simulink model "IRSensor"  (Simulink 8.7)
settings: Solver=VariableStepAuto  StartTime=0.0  StopTime=10.0  RelTol=1e-3
settings Model: Creator=maximilian  LastModifiedBy=maximilian
settings DataIOCC: LimitDataPoints=off  SaveFormat=Dataset
settings DebuggingCC: UnderspecifiedInitializationDetection=Simplified  MergeDetectMultiDrivingBlocksExec=error
settings HardwareCC: ProdBitPerPointer=64  ProdLargestAtomicFloat=Float  ProdIntDivRoundTo=Zero  ProdEndianess=LittleEndian  ProdWordSize=64  ProdHWDeviceType=Intel->x86-64 (Windows64)
settings ModelReferenceCC: PropagateSignalLabelsOutOfModel=on
settings ConfigComp: CovModelRefEnable=off

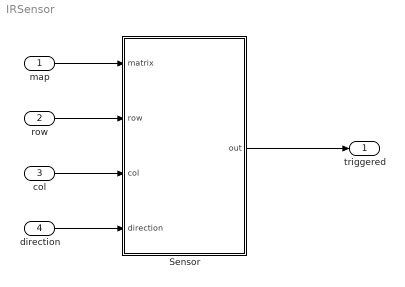
== system IRSensor ==
  map : Inport  PortDimensions=[100 100]
  row : Inport  Port=2
  col : Inport  Port=3
  direction : Inport  Port=4
  Sensor : MATLAB Function  TreatAsAtomicUnit=on
  triggered : Outport
  wires:
  map/1 -> Sensor/1(matrix)
  col/1 -> Sensor/3(col)
  row/1 -> Sensor/2(row)
  direction/1 -> Sensor/4(direction)
  Sensor/1(out) -> triggered/1

== matlab function Sensor ==
  data: matrix input double; row input double; col input double; out output double; direction input double
function out  = raycast(matrix, row, col, direction)
    out = 0;
    start = mod(direction - deg2rad(80) / 2, 2 * pi);
    step = deg2rad(80) / 100;
    for i = 0:100
        [~, object] = TinUtils.raycast(matrix, row, col, start + step * i);
        if (object == 2)
            out = 1;
            break;
        end
    end
end
